simulink model "LETS_GOOOOOO"  (R2020b)
settings: Solver=VariableStepAuto  StartTime=0.0  StopTime=60  RelTol=1e-3
values from neighbouring files (symbols this model uses):
  A_2 = zeros(3)    [MPC_tune.m]
  B_2 = I_inv    [MPC_tune.m]
  C_2 = eye(3)    [MPC_tune.m]
  D_2 = zeros(3)    [MPC_tune.m]
  I_inv = inv(I_mat)    [MPC_tune.m]
  m = 941.102    [Linear_tuning.m]
  TcgCatia = [1 0 0 ... (first row only)    [MPC_tune.m]
undefined symbols (not defined in the file or in its folder): A_kal, B_kal, C_kal, Continuous, D_kal, delta_time, F_tot_max, Fb1_l, Fb1_u, Fb2_l, Fb2_u, Fb3_l, Fb3_u, Fb4_l, Fb4_u, Fc1_l, Fc1_u, Fc2_l, Fc2_u, Fc3_l, Fc3_u, fprop, Ft1_l, Ft1_u, Ft2_l, Ft2_u, Ft3_l, Ft3_u, Ft4_l, Ft4_u, g, r_0, r_cgCatia, r_trajectory, rho, T, t_finalgust, theta0, time, Time, time_delay, Tzy_Shard, u0_final, u0_ini, u1_final, u1_ini, u2_final, u2_ini, u_0, u_1, u_2, v_0, ZI_Cx, ZI_Cy, ZI_Cz, ZI_p, ZI_q, ZI_r
libraries: dspsigops x11, simulink x6, pid_lib x6, fuzblock x3, sharedutil x1, mpclib x1, dspmathops x1, ctrlSharedLib x1
(part 1 of 2)
settings Model: Creator=Jonathan van Zyl  LastModifiedBy=Jonathan van Zyl

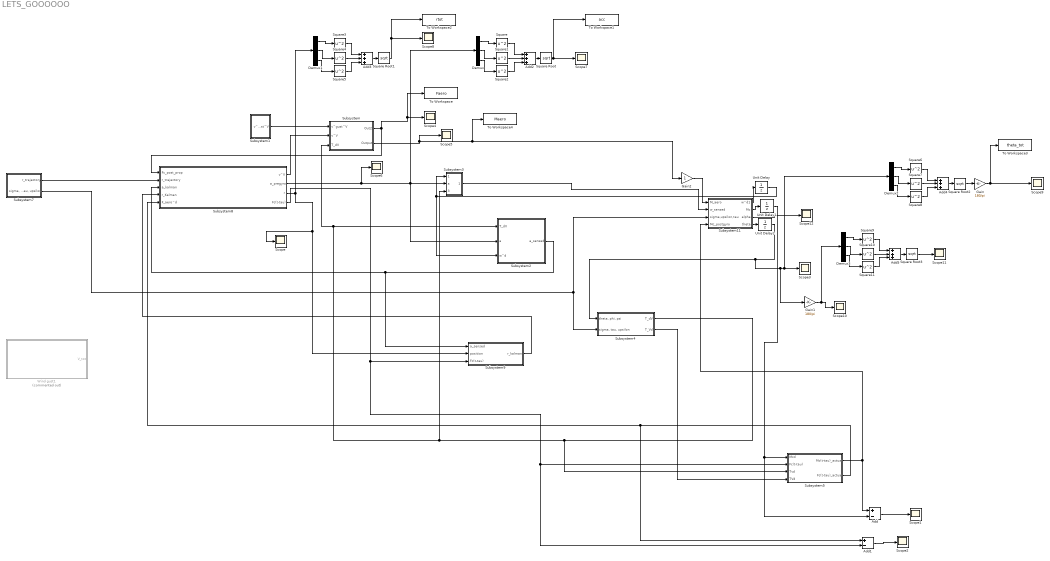
== system LETS_GOOOOOO ==
  Add : Sum  Inputs=+-
  Add1 : Sum  Inputs=+-
  Add{2..5} (4 alike) : Sum  Inputs=+++
  Demux{,1..3} (4 alike) : Demux  Outputs=3
  Gain : Gain  Gain=180/pi
  Gain1 : Gain  Gain=180/pi
  Gain2 : Gain
  Scope{,1..12} (13 alike) : Scope
  Square{,1..11} (12 alike) : Math  Operator=square  SaturateOnIntegerOverflow=on
  Square Root{,1..3} (4 alike) : Sqrt  SaturateOnIntegerOverflow=on
  Subsystem : Subsystem
  Subsystem1 : Subsystem
  Subsystem11 : Subsystem
  Subsystem2 : Subsystem
  Subsystem3 : Subsystem
  Subsystem4 : Subsystem
  Subsystem5 : Subsystem
  Subsystem7 : Subsystem
  Subsystem8 : Subsystem
  Subsystem9 : Subsystem
  To Workspace : ToWorkspace  VariableName=Faero  SaveFormat=Timeseries  SampleTime=-1
  To Workspace1 : ToWorkspace  VariableName=acc  SaveFormat=Timeseries  SampleTime=-1
  To Workspace2 : ToWorkspace  VariableName=rtot  SaveFormat=Timeseries  SampleTime=-1
  To Workspace3 : ToWorkspace  VariableName=theta_tot  SaveFormat=Timeseries  SampleTime=-1
  To Workspace4 : ToWorkspace  VariableName=Maero  SaveFormat=Timeseries  SampleTime=-1
  Unit Delay : UnitDelay  SampleTime=-1  HasFrameUpgradeWarning=on
  Unit Delay1 : UnitDelay  SampleTime=-1  HasFrameUpgradeWarning=on
  Unit Delay2 : UnitDelay  SampleTime=-1  HasFrameUpgradeWarning=on
  Wind gust1 : Subsystem  Commented=on
  wires:
  Unit Delay2/1 -> Gain1/1, Demux2/1, Scope3/1, Subsystem4/1("theta, phi, psi")
  Square9/1 -> Add5/1
  Subsystem/1(Out2) -> To Workspace/1, Scope4/1, Subsystem8/1(Fc_post_prop)
  Square1/1 -> Add2/2
  Subsystem/2(Output) -> Scope5/1, Gain2/1, To Workspace4/1
  Demux3/1 -> Square9/1
  Subsystem5/2(Fc(t-tau)_actual) -> Add1/1, Subsystem8/5(F_aero^d)
  Subsystem4/2(T_Vd) -> Subsystem5/4(TVd)
  Demux2/3 -> Square8/1
  Add1/1 -> Scope2/1
  Demux/3 -> Square2/1
  Square Root1/1 -> To Workspace2/1, Scope8/1
  Subsystem7/1(r_trajectory) -> Subsystem8/2(r_trajectory)
  Demux1/3 -> Square5/1
  Subsystem11/3(alpha) -> Scope12/1
  Demux2/2 -> Square7/1
  Subsystem8/2(a_pregyro) -> Scope6/1, Demux/1, Subsystem3/2(a), Subsystem2/2(a)
  Square10/1 -> Add5/2
  Add2/1 -> Square Root/1
  Subsystem5/1(Mc(t-tau)_actual) -> Subsystem11/4(Mc_postgyro), Add/1
  Demux/1 -> Square/1
  Square Root/1 -> To Workspace1/1, Scope7/1
  Subsystem7/2("sigma, tau, upsilon") -> Subsystem11/3(sigma,upsilon,tau), Subsystem4/2("sigma, tau, upsilon")
  Square4/1 -> Add3/2
  Subsystem4/1(T_dV) -> Subsystem5/3(Tvd), Subsystem/3(T_dV), Subsystem2/1(T_dV), Subsystem3/3(T_dV)
  Add4/1 -> Square Root2/1
  Unit Delay/1 -> Subsystem2/3(w^d), Subsystem3/1(w^d)
  Gain/1 -> To Workspace3/1, Scope9/1
  Demux2/1 -> Square6/1
  Subsystem2/1(a_sensed) -> Subsystem8/3(a_kalman), Subsystem9/1(a_sensed)
  Subsystem9/1(r_kalman) -> Subsystem8/4(r_Kalman)
  Square/1 -> Add2/1
  Square5/1 -> Add3/3
  Add/1 -> Scope1/1
  Demux/2 -> Square1/1
  Square6/1 -> Add4/1
  Square Root2/1 -> Gain/1
  Demux1/2 -> Square4/1
  Unit Delay1/1 -> Add/2, Subsystem5/1(Mcd)
  Square3/1 -> Add3/1
  Add3/1 -> Square Root1/1
  Subsystem8/3(r) -> Scope/1, Subsystem9/2(position), Demux1/1
  Demux1/1 -> Square3/1
  Square8/1 -> Add4/3
  Gain1/1 -> Demux3/1, Scope10/1
  Gain2/1 -> Subsystem11/1(M_aero)
  Demux3/2 -> Square10/1
  Subsystem8/1(v^V) -> Subsystem/2(v^V)
  Subsystem8/4(Fc(t-tau)) -> Add1/2, Subsystem5/2(Fc(t-tau)), Subsystem9/3(Fc(t-tau))
  Square7/1 -> Add4/2
  Square2/1 -> Add2/3
  Subsystem3/1(w^d1) -> Subsystem11/2(w_sensed)
  Add5/1 -> Square Root3/1
  Subsystem1/1(v^gust^V) -> Subsystem/1(v^gust^V)
  Square11/1 -> Add5/3
  Square Root3/1 -> Scope11/1
  Demux3/3 -> Square11/1
  Subsystem11/1(w^d1) -> Unit Delay/1
  Subsystem11/2(Mc) -> Unit Delay1/1
  Subsystem11/4(theta) -> Unit Delay2/1

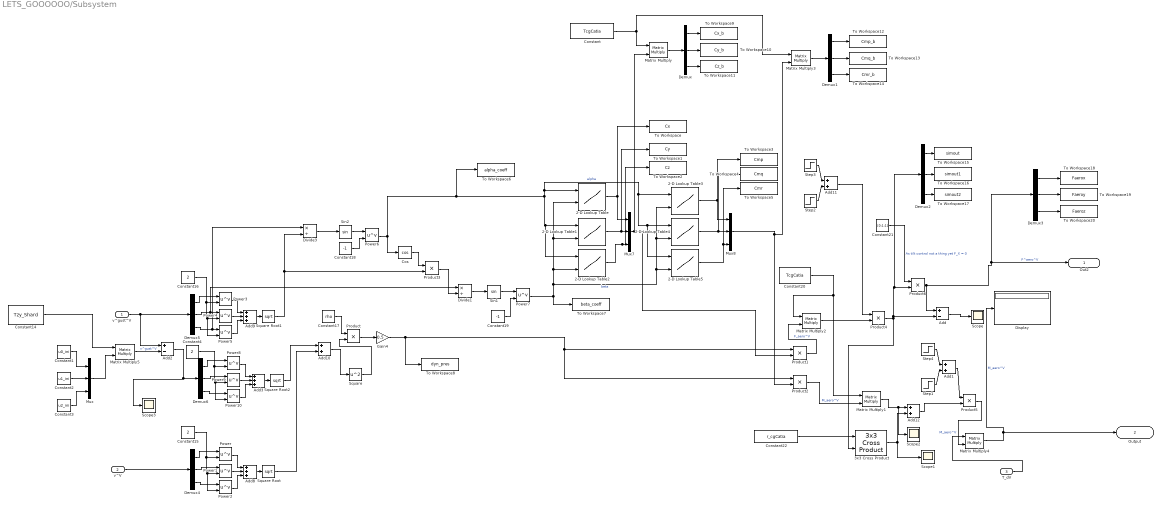
== system LETS_GOOOOOO/Subsystem ==
  v^gust^V : Inport
  v^V : Inport  Port=2
  T_dV : Inport  Port=3
  2-D Lookup Table : Lookup_n-D  BreakpointsForDimension1=[-180:1:180]  BreakpointsForDimension2=[-90:1:90]  Table=ZI_Cx  InternalRulePriority=Speed  RndMeth=Simplest  InputSameDT=on
      settings: InputPortMap=u0,u1
  2-D Lookup Table1 : Lookup_n-D  BreakpointsForDimension1=[-180:1:180]  BreakpointsForDimension2=[-90:1:90]  Table=ZI_Cy  InternalRulePriority=Speed  RndMeth=Simplest  InputSameDT=on
      settings: InputPortMap=u0,u1
  2-D Lookup Table2 : Lookup_n-D  BreakpointsForDimension1=[-180:1:180]  BreakpointsForDimension2=[-90:1:90]  Table=ZI_Cz  InternalRulePriority=Speed  RndMeth=Simplest  InputSameDT=on
      settings: InputPortMap=u0,u1
  2-D Lookup Table3 : Lookup_n-D  BreakpointsForDimension1=[-180:1:180]  BreakpointsForDimension2=[-90:1:90]  Table=ZI_p  InternalRulePriority=Speed  RndMeth=Simplest  InputSameDT=on
      settings: InputPortMap=u0,u1
  2-D Lookup Table4 : Lookup_n-D  BreakpointsForDimension1=[-180:1:180]  BreakpointsForDimension2=[-90:1:90]  Table=ZI_q  InternalRulePriority=Speed  RndMeth=Simplest  InputSameDT=on
      settings: InputPortMap=u0,u1
  2-D Lookup Table5 : Lookup_n-D  BreakpointsForDimension1=[-180:1:180]  BreakpointsForDimension2=[-90:1:90]  Table=ZI_r  InternalRulePriority=Speed  RndMeth=Simplest  InputSameDT=on
      settings: InputPortMap=u0,u1
  3x3 Cross Product : sharedutil/3x3 Cross Product  aMode=aMode
      settings: SourceProductBaseCode=AE,PW,MT,UV,VE,VP
  Add : Sum  Inputs=+-
  Add{1,10..12} (4 alike) : Sum
  Add2 : Sum  Inputs=+-
  Add3 : Sum  Inputs=+++
  Add8 : Sum  Inputs=+++
  Add9 : Sum  Inputs=+++
  Constant : Constant  Value=TcgCatia
  Constant1 : Constant  Value=u0_ini
  Constant14 : Constant  Value=Tzy_Shard
  Constant15 : Constant  Value=2
  Constant16 : Constant  Value=2
  Constant17 : Constant  Value=rho
  Constant18 : Constant  Value=-1
  Constant19 : Constant  Value=-1
  Constant2 : Constant  Value=u1_ini
  Constant20 : Constant  Value=TcgCatia
  Constant21 : Constant  Value=[0;1;1]
  Constant22 : Constant  Value=r_cgCatia
  Constant3 : Constant  Value=u2_ini
  Constant4 : Constant  Value=2
  Cos : Trigonometry  Operator=cos
  Demux{,1..6} (7 alike) : Demux  Outputs=3
  Display : Display
  Divide1 : Product  Inputs=*/
  Divide3 : Product  Inputs=*/
  Gain4 : Gain  Gain=0.5
  Matrix Multiply{,1..5} (6 alike) : Product  Multiplication=Matrix(*)
  Mux : Mux  Inputs=3
  Mux7 : Mux  Inputs=3
  Mux8 : Mux  Inputs=3
  Power{,1..10} (11 alike) : Math  Operator=pow  SaturateOnIntegerOverflow=on
  Product{,1..6} (7 alike) : Product
  Scope{,1..3} (4 alike) : Scope
  Sin1 : Trigonometry
  Sin2 : Trigonometry
  Square : Math  Operator=square  SaturateOnIntegerOverflow=on
  Square Root : Sqrt  SaturateOnIntegerOverflow=on
  Square Root1 : Sqrt  SaturateOnIntegerOverflow=on
  Square Root2 : Sqrt  SaturateOnIntegerOverflow=on
  Step1 : Step  Time=0  SampleTime=0
  Step2 : Step  Time=0  SampleTime=0
  Step3 : Step  Time=time  After=-1  SampleTime=0
  Step4 : Step  Time=time  After=-1  SampleTime=0
  To Workspace : ToWorkspace  VariableName=Cx  SaveFormat=Timeseries  SampleTime=-1
  To Workspace1 : ToWorkspace  VariableName=Cy  SaveFormat=Timeseries  SampleTime=-1
  To Workspace10 : ToWorkspace  VariableName=Cy_b  SaveFormat=Timeseries  SampleTime=-1
  To Workspace11 : ToWorkspace  VariableName=Cz_b  SaveFormat=Timeseries  SampleTime=-1
  To Workspace12 : ToWorkspace  VariableName=Cmp_b  SaveFormat=Timeseries  SampleTime=-1
  To Workspace13 : ToWorkspace  VariableName=Cmq_b  SaveFormat=Timeseries  SampleTime=-1
  To Workspace14 : ToWorkspace  VariableName=Cmr_b  SaveFormat=Timeseries  SampleTime=-1
  To Workspace15 : ToWorkspace  VariableName=simout  SaveFormat=Timeseries  SampleTime=-1
  To Workspace16 : ToWorkspace  VariableName=simout1  SaveFormat=Timeseries  SampleTime=-1
  To Workspace17 : ToWorkspace  VariableName=simout2  SaveFormat=Timeseries  SampleTime=-1
  To Workspace18 : ToWorkspace  VariableName=Faerox  SaveFormat=Timeseries  SampleTime=-1
  To Workspace19 : ToWorkspace  VariableName=Faeroy  SaveFormat=Timeseries  SampleTime=-1
  To Workspace2 : ToWorkspace  VariableName=Cz  SaveFormat=Timeseries  SampleTime=-1
  To Workspace20 : ToWorkspace  VariableName=Faeroz  SaveFormat=Timeseries  SampleTime=-1
  To Workspace3 : ToWorkspace  VariableName=Cmp  SaveFormat=Timeseries  SampleTime=-1
  To Workspace4 : ToWorkspace  VariableName=Cmq  SaveFormat=Timeseries  SampleTime=-1
  To Workspace5 : ToWorkspace  VariableName=Cmr  SaveFormat=Timeseries  SampleTime=-1
  To Workspace6 : ToWorkspace  VariableName=alpha_coeff  SaveFormat=Timeseries  SampleTime=-1
  To Workspace7 : ToWorkspace  VariableName=beta_coeff  SaveFormat=Timeseries  SampleTime=-1
  To Workspace8 : ToWorkspace  VariableName=dyn_pres  SaveFormat=Timeseries  SampleTime=-1
  To Workspace9 : ToWorkspace  VariableName=Cx_b  SaveFormat=Timeseries  SampleTime=-1
  Out2 : Outport
  Output : Outport  Port=2
  wires:
  Demux5/1 -> Power3/1
  Constant21/1 -> Product6/1  "As tilt control not a thing yet F_X = 0"
  2-D Lookup Table3/1 -> To Workspace3/1, Mux8/1
  Constant17/1 -> Product/1
  Power5/1 -> Add9/3
  Product4/1 -> Demux2/1, Product6/2, Add/2, 3x3 Cross Product/2
  Power7/1 -> 2-D Lookup Table/2, 2-D Lookup Table1/2, 2-D Lookup Table2/2, 2-D Lookup Table3/2, 2-D Lookup Table4/2, 2-D Lookup Table5/2, To Workspace7/1  "beta"
  2-D Lookup Table2/1 -> To Workspace2/1, Mux7/3
  Power3/1 -> Add9/1
  Constant15/1 -> Power2/2, Power1/2, Power/2
  Sin1/1 -> Power7/1
  Square/1 -> Product/2
  Demux4/2 -> Power1/1
  Gain4/1 -> To Workspace8/1, Product2/1, Product1/1
  Square Root1/1 -> Product3/2, Divide3/2
  Product1/1 -> Matrix Multiply2/2  "F_aero^V"
  2-D Lookup Table1/1 -> To Workspace1/1, Mux7/2
  Add8/1 -> Square Root/1
  Cos/1 -> Product3/1
  3x3 Cross Product/1 -> Add12/2, Scope1/1
  Power2/1 -> Add8/3
  Add9/1 -> Square Root1/1
  Divide3/1 -> Sin2/1
  Mux7/1 -> Matrix Multiply/2, Product1/2
  Demux5/2 -> Divide1/1, Power4/1
  Product3/1 -> Divide1/2
  Constant22/1 -> 3x3 Cross Product/1
  Product2/1 -> Matrix Multiply1/2  "M_aero^V"
  Demux4/3 -> Power2/1
  Square Root/1 -> Add10/2
  Constant16/1 -> Power5/2, Power4/2, Power3/2
  2-D Lookup Table5/1 -> To Workspace5/1, Mux8/3
  v^gust^V/1 -> Add2/1, Demux5/1
  Divide1/1 -> Sin1/1
  Power1/1 -> Add8/2
  Constant20/1 -> Matrix Multiply1/1, Matrix Multiply2/1
  Power4/1 -> Add9/2
  Power/1 -> Add8/1
  2-D Lookup Table4/1 -> To Workspace4/1, Mux8/2
  Matrix Multiply1/1 -> Scope2/1, Add12/1
  Mux8/1 -> Matrix Multiply3/2, Product2/2
  Constant18/1 -> Power6/2
  Demux4/1 -> Power/1
  Product6/1 -> Add/1, Out2/1, Demux3/1  "F^aero^V"
  Demux5/3 -> Divide3/1, Power5/1
  Product/1 -> Gain4/1
  Power6/1 -> Cos/1, To Workspace6/1, 2-D Lookup Table/1, 2-D Lookup Table5/1, 2-D Lookup Table4/1, 2-D Lookup Table3/1, 2-D Lookup Table2/1, 2-D Lookup Table1/1  "alpha"
  Sin2/1 -> Power6/1
  Constant19/1 -> Power7/2
  2-D Lookup Table/1 -> Mux7/1, To Workspace/1
  Add10/1 -> Square/1
  Matrix Multiply4/1 -> Display/1, Output/1  "M_aero^V"
  T_dV/1 -> Matrix Multiply4/1
  v^V/1 -> Demux4/1
  Add/1 -> Scope/1
  Constant/1 -> Matrix Multiply3/1, Matrix Multiply/1
  Matrix Multiply/1 -> Demux/1
  Demux/1 -> To Workspace9/1
  Demux/2 -> To Workspace10/1
  Demux/3 -> To Workspace11/1
  Matrix Multiply3/1 -> Demux1/1
  Demux1/1 -> To Workspace12/1
  Demux1/2 -> To Workspace13/1
  Demux1/3 -> To Workspace14/1
  Demux2/1 -> To Workspace15/1
  Demux2/2 -> To Workspace16/1
  Demux2/3 -> To Workspace17/1
  Demux3/1 -> To Workspace18/1
  Demux3/2 -> To Workspace19/1
  Demux3/3 -> To Workspace20/1
  Step3/1 -> Add11/1
  Add11/1 -> Product4/1
  Step2/1 -> Add11/2
  Matrix Multiply2/1 -> Product4/2
  Add1/1 -> Product5/1
  Step1/1 -> Add1/2
  Step4/1 -> Add1/1
  Product5/1 -> Matrix Multiply4/2  "M_aero^V"
  Add12/1 -> Product5/2
  Mux/1 -> Matrix Multiply5/2
  Constant3/1 -> Mux/3
  Constant1/1 -> Mux/1
  Constant2/1 -> Mux/2
  Add2/1 -> Demux6/1, Scope3/1
  Constant14/1 -> Matrix Multiply5/1
  Matrix Multiply5/1 -> Add2/2  "v^gust^V"
  Power10/1 -> Add3/3
  Demux6/3 -> Power10/1
  Add3/1 -> Square Root2/1
  Power9/1 -> Add3/2
  Power8/1 -> Add3/1
  Demux6/2 -> Power9/1
  Demux6/1 -> Power8/1
  Square Root2/1 -> Add10/1
  Constant4/1 -> Power8/2, Power9/2, Power10/2

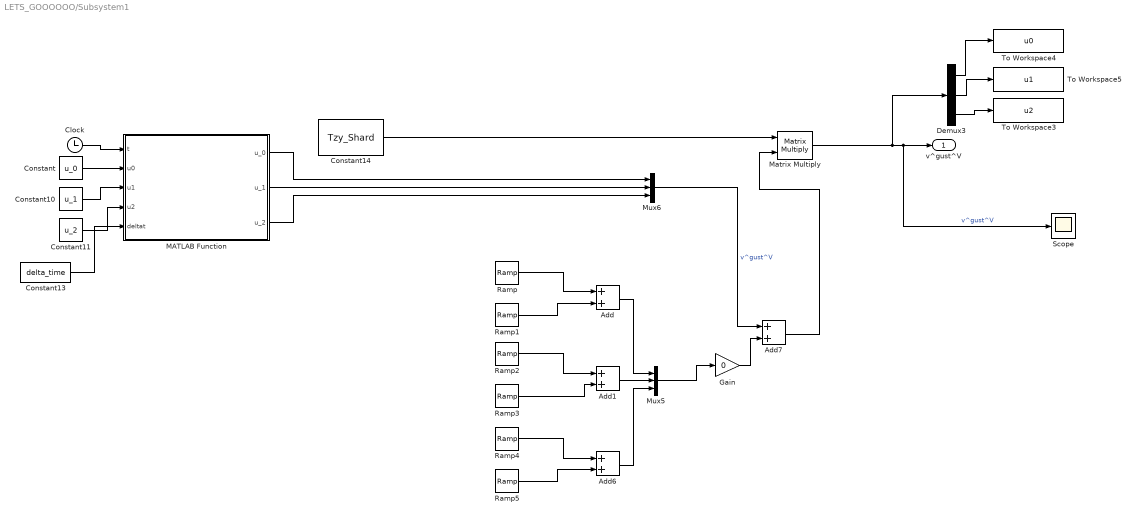
== system LETS_GOOOOOO/Subsystem1 ==
  Add{,1,6..7} (4 alike) : Sum
  Clock : Clock
  Constant : Constant  Value=u_0
  Constant10 : Constant  Value=u_1
  Constant11 : Constant  Value=u_2
  Constant13 : Constant  Value=delta_time
  Constant14 : Constant  Value=Tzy_Shard
  Demux3 : Demux  Outputs=3
  Gain : Gain  Gain=0
  MATLAB Function : MATLAB Function  TreatAsAtomicUnit=on
  Matrix Multiply : Product  Multiplication=Matrix(*)
  Mux5 : Mux  Inputs=3
  Mux6 : Mux  Inputs=3
  Ramp : simulink/Sources/Ramp  slope=-1  start=t_finalgust  InitialOutput=0
  Ramp1 : simulink/Sources/Ramp  slope=1  start=t_finalgust + u0_final  InitialOutput=0
  Ramp2 : simulink/Sources/Ramp  slope=-1  start=t_finalgust  InitialOutput=0
  Ramp3 : simulink/Sources/Ramp  slope=1  start=t_finalgust + u1_final  InitialOutput=0
  Ramp4 : simulink/Sources/Ramp  slope=-1  start=t_finalgust  InitialOutput=0
  Ramp5 : simulink/Sources/Ramp  slope=1  start=t_finalgust + u2_final  InitialOutput=0
  Scope : Scope
  To Workspace3 : ToWorkspace  VariableName=u2  SaveFormat=Timeseries  SampleTime=-1
  To Workspace4 : ToWorkspace  VariableName=u0  SaveFormat=Timeseries  SampleTime=-1
  To Workspace5 : ToWorkspace  VariableName=u1  SaveFormat=Timeseries  SampleTime=-1
  v^gust^V : Outport
  wires:
  Add1/1 -> Mux5/2
  MATLAB Function/1(u_0) -> Mux6/1
  Add7/1 -> Matrix Multiply/2
  Constant13/1 -> MATLAB Function/5(deltat)
  Ramp4/1 -> Add6/1
  Ramp3/1 -> Add1/2
  Constant11/1 -> MATLAB Function/4(u2)
  Constant/1 -> MATLAB Function/2(u0)
  Ramp1/1 -> Add/2
  Mux5/1 -> Gain/1
  Constant14/1 -> Matrix Multiply/1
  MATLAB Function/2(u_1) -> Mux6/2
  Constant10/1 -> MATLAB Function/3(u1)
  Ramp/1 -> Add/1
  Matrix Multiply/1 -> Demux3/1, Scope/1, v^gust^V/1  "v^gust^V"
  Ramp5/1 -> Add6/2
  Add6/1 -> Mux5/3
  Clock/1 -> MATLAB Function/1(t)
  MATLAB Function/3(u_2) -> Mux6/3
  Add/1 -> Mux5/1
  Ramp2/1 -> Add1/1
  Mux6/1 -> Add7/1  "v^gust^V"
  Demux3/3 -> To Workspace3/1
  Demux3/2 -> To Workspace5/1
  Demux3/1 -> To Workspace4/1
  Gain/1 -> Add7/2

== system LETS_GOOOOOO/Subsystem11 ==
  M_aero : Inport
  w_sensed : Inport  Port=2
  sigma,upsilon,tau : Inport  Port=3
  Mc_postgyro : Inport  Port=4
  Add : Sum  Inputs=+++
  Demux : Demux  Outputs=3
  Gain3 : Gain  Gain=180/pi
  Scope : Scope
  Scope1 : Scope
  Scope8 : Scope
  Square : Math  Operator=square  SaturateOnIntegerOverflow=on
  Square Root : Sqrt  SaturateOnIntegerOverflow=on
  Square1 : Math  Operator=square  SaturateOnIntegerOverflow=on
  Square2 : Math  Operator=square  SaturateOnIntegerOverflow=on
  Subsystem : Subsystem
  To Workspace : ToWorkspace  VariableName=angle_deg  SaveFormat=Timeseries  SampleTime=-1
  To Workspace1 : ToWorkspace  VariableName=alpha  SaveFormat=Timeseries  SampleTime=-1
  initial w : Constant  Value=[0;0;0]
  w^d1 : Outport
  Mc : Outport  Port=2
  alpha : Outport  Port=3
  theta : Outport  Port=4
  wires:
  Mc_postgyro/1 -> Subsystem/5(Mcpost)
  Subsystem/4(alpha) -> Demux/1, Scope/1, alpha/1
  Demux/1 -> Square/1
  Demux/2 -> Square1/1
  Demux/3 -> Square2/1
  Square/1 -> Add/1
  Square1/1 -> Add/2
  Square2/1 -> Add/3
  Add/1 -> Square Root/1
  Square Root/1 -> To Workspace1/1, Scope1/1
  sigma,upsilon,tau/1 -> Subsystem/3(sigma,tau,upsilon)
  initial w/1 -> Subsystem/4(initial w)
  M_aero/1 -> Subsystem/2(M_aero)
  Subsystem/3(Mc) -> Mc/1
  Subsystem/2(w_out) -> w^d1/1
  Subsystem/1(theta_out) -> Gain3/1, theta/1
  Gain3/1 -> To Workspace/1, Scope8/1
  w_sensed/1 -> Subsystem/1(w_sensed)

== system LETS_GOOOOOO/Subsystem2 ==
  T_dV : Inport
  a : Inport  Port=2
  w^d : Inport  Port=3
  Display1 : Display
  Display2 : Display
  MATLAB Function1 : MATLAB Function  Commented=on  TreatAsAtomicUnit=on
  Terminator5 : Terminator
  Terminator6 : Terminator
  Transpose1 : Math  Operator=transpose  SaturateOnIntegerOverflow=on
  Transpose2 : Math  Operator=transpose  SaturateOnIntegerOverflow=on
  Transpose3 : Math  Operator=transpose  SaturateOnIntegerOverflow=on
  a_sensed : Outport
  wires:
  a/1 -> Transpose1/1
  Transpose1/1 -> Display1/1, Transpose2/1, Display2/1  "a_sensed"
  Transpose3/1 -> Terminator5/1
  T_dV/1 -> Terminator6/1
  Transpose2/1 -> a_sensed/1  "a_sensed"
  w^d/1 -> Transpose3/1

== system LETS_GOOOOOO/Subsystem3 ==
  w^d : Inport
  a : Inport  Port=2
  T_dV : Inport  Port=3
  Add : Sum  Inputs=+-
  Add1 : Sum
  Demux21 : Demux  Outputs=3
  Demux22 : Demux  Outputs=3
  Gain : Gain  Gain=0
  Gain1 : Gain
  MATLAB Function10 : MATLAB Function  TreatAsAtomicUnit=on
  Matrix Multiply4 : Product  Multiplication=Matrix(*)
  Mux14 : Mux  Inputs=3
  To Workspace : ToWorkspace  VariableName=gyro  SaveFormat=Timeseries  SampleTime=-1
  w^d1 : Outport
  wires:
  Demux21/3 -> MATLAB Function10/3(zvel)
  Demux22/1 -> MATLAB Function10/4(accx)
  Demux22/2 -> MATLAB Function10/5(accy)
  Demux22/3 -> MATLAB Function10/6(accz)
  MATLAB Function10/1(wx) -> Mux14/1
  Demux21/1 -> MATLAB Function10/1(xvel)
  MATLAB Function10/2(wy) -> Mux14/2
  Demux21/2 -> MATLAB Function10/2(yvel)
  MATLAB Function10/3(wz) -> Mux14/3
  Matrix Multiply4/1 -> Demux22/1
  Mux14/1 -> Gain/1, Add/2  "w^d"
  T_dV/1 -> Matrix Multiply4/1
  a/1 -> Matrix Multiply4/2
  w^d/1 -> Gain1/1, Add/1, Demux21/1
  Add/1 -> To Workspace/1
  Gain/1 -> Add1/1
  Gain1/1 -> Add1/2
  Add1/1 -> w^d1/1

== system LETS_GOOOOOO/Subsystem4 ==
  "theta, phi, psi" : Inport
  "sigma, tau, upsilon" : Inport  Port=2
  Demux6 : Demux  Outputs=3
  Demux7 : Demux  Outputs=3
  MATLAB Function2 : MATLAB Function  TreatAsAtomicUnit=on
  MATLAB Function3 : MATLAB Function  TreatAsAtomicUnit=on
  Matrix Multiply7 : Product  Multiplication=Matrix(*)
  Terminator{7..10} (4 alike) : Terminator
  Transpose4 : Math  Operator=transpose  SaturateOnIntegerOverflow=on
  Transpose5 : Math  Operator=transpose  SaturateOnIntegerOverflow=on
  Transpose6 : Math  Operator=transpose  SaturateOnIntegerOverflow=on
  T_dV : Outport
  T_Vd : Outport  Port=2
  wires:
  Matrix Multiply7/1 -> T_Vd/1, Transpose6/1  "T_Vd"
  Demux7/1 -> MATLAB Function3/1(theta_x)
  "theta, phi, psi"/1 -> Demux6/1
  Demux6/3 -> MATLAB Function2/3(theta_z)
  Demux7/3 -> MATLAB Function3/3(theta_z)
  "sigma, tau, upsilon"/1 -> Demux7/1
  Demux6/1 -> MATLAB Function2/1(theta_x)
  Transpose5/1 -> Terminator9/1, Matrix Multiply7/2  "T_Vt"
  MATLAB Function2/1(Transformation_Mat) -> Terminator7/1, Transpose4/1  "T_dt"
  Transpose4/1 -> Terminator8/1, Matrix Multiply7/1  "T_td"
  MATLAB Function3/1(Transformation_Mat) -> Terminator10/1, Transpose5/1  "T_tV"
  Demux6/2 -> MATLAB Function2/2(theta_y)
  Demux7/2 -> MATLAB Function3/2(theta_y)
  Transpose6/1 -> T_dV/1  "T_dV"

== system LETS_GOOOOOO/Subsystem5 ==
  Mcd : Inport
  Fc(t-tau) : Inport  Port=2
  Tvd : Inport  Port=3
  TVd : Inport  Port=4
  Gain6 : Gain
  MATLAB Function4 : MATLAB Function  Commented=on  TreatAsAtomicUnit=on
  MATLAB Function5 : MATLAB Function  Commented=on  TreatAsAtomicUnit=on
  Matrix Multiply5 : Product  Multiplication=Matrix(*)
  Scope16 : Scope
  Scope17 : Scope
  Scope18 : Scope
  Subsystem : Subsystem
  Subsystem1 : Subsystem
  Subsystem2 : Subsystem
  Subsystem3 : Subsystem
  Subsystem4 : Subsystem
  Turn off for PID tune : Gain
  Mc(t-tau)_actual : Outport
  Fc(t-tau)_actual : Outport  Port=2
  wires:
  Mcd/1 -> Gain6/1
  Turn off for PID tune/1 -> Matrix Multiply5/2
  Tvd/1 -> Matrix Multiply5/1
  Fc(t-tau)/1 -> Turn off for PID tune/1
  MATLAB Function5/1(F1) -> MATLAB Function4/1(F1)
  MATLAB Function5/3(F3) -> MATLAB Function4/3(F3)
  MATLAB Function5/2(F2) -> MATLAB Function4/2(F2)
  Matrix Multiply5/1 -> Subsystem/1(F_c_d)  "F_c_d"
  Gain6/1 -> Subsystem/2(M_c_d)  "M_c_d"
  Subsystem/1(Fb_wanted) -> Subsystem1/1(In1)
  Subsystem/2(Ft_wanted) -> Subsystem1/2(In2)
  Subsystem/3(Fc_wanted) -> Subsystem1/3(In3)
  Subsystem1/1(Out1) -> Subsystem2/1(In1)
  Subsystem1/2(Out2) -> Subsystem2/2(In2)
  Subsystem1/3(Out3) -> Subsystem2/3(In3)
  Subsystem3/1(Out1) -> Scope17/1, Subsystem4/2(In2)
  Subsystem2/1(F_c_max) -> Subsystem3/1(In1)
  Subsystem2/2(F_t_max) -> Subsystem3/2(In2)
  Subsystem2/3(Out3) -> Subsystem3/3(In3)
  Subsystem2/4(Out4) -> Subsystem3/4(Ft3)
  Subsystem2/5(Out5) -> Subsystem3/5(Ft4)
  Subsystem2/6(Out6) -> Subsystem3/6(Fb1)
  Subsystem2/7(Out7) -> Subsystem3/7(In7)
  Subsystem2/8(Out8) -> Subsystem3/8(Fb3)
  Subsystem2/9(Out9) -> Subsystem3/9(In9)
  Subsystem3/2(Mc(t-tau)_actual) -> Mc(t-tau)_actual/1
  Subsystem4/1(Fc(t-tau)_actual) -> Scope16/1, Fc(t-tau)_actual/1
  TVd/1 -> Subsystem4/1(TVd)
  Subsystem4/2(Fc(t-tau)_actual1) -> Scope18/1

== system LETS_GOOOOOO/Subsystem7 ==
  Constant2 : Constant  Value=r_trajectory
  Constant9 : Constant  Value=[0;0;0]
  r_trajectory : Outport
  "sigma, tau, upsilon" : Outport  Port=2
  wires:
  Constant2/1 -> r_trajectory/1
  Constant9/1 -> "sigma, tau, upsilon"/1  "sigma, tau, upsilon"

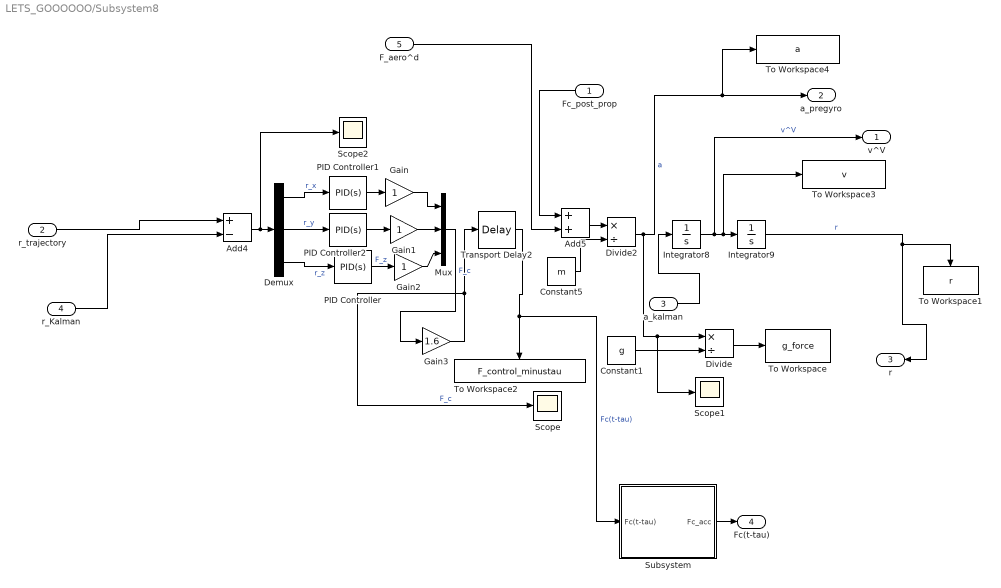
== system LETS_GOOOOOO/Subsystem8 ==
  Fc_post_prop : Inport
  r_trajectory : Inport  Port=2
  a_kalman : Inport  Port=3
  r_Kalman : Inport  Port=4
  F_aero^d : Inport  Port=5
  Add4 : Sum  Inputs=+-
  Add5 : Sum
  Constant1 : Constant  Value=g
  Constant5 : Constant  Value=m
  Demux : Demux  Outputs=3
  Divide : Product  Inputs=*/
  Divide2 : Product  Inputs=*/
  Gain : Gain
  Gain1 : Gain
  Gain2 : Gain
  Gain3 : Gain  Gain=1.6
  Integrator8 : Integrator  InitialCondition=v_0
  Integrator9 : Integrator  InitialCondition=r_0
  Mux : Mux  Inputs=3
  PID Controller : pid_lib/PID Controller  Controller=PID  Form=Parallel  TimeDomain=Continuous-time  UseExternalTs=off  SampleTime=-1  IntegratorMethod=Forward Euler  FilterMethod=Forward Euler  ControllerParametersSource=internal  P=160.734193661502  I=6.85755125615993  D=923.025793270617  UseFilter=on  N=10.4897155810233  TunerSelectOption=Transfer Function Based (PID Tuner App)  InitialConditionSource=internal  InitialConditionForIntegrator=0  InitialConditionForFilter=0  DifferentiatorICPrevScaledInput=0  ExternalReset=none  TrackingMode=off  Kt=1  LimitOutput=off  SatLimitsSource=internal  UpperSaturationLimit=inf  LowerSaturationLimit=-inf  LinearizeAsGain=on  AntiWindupMode=none  Kb=1  POutMin=[]  POutMax=[]  IOutMin=[]  IOutMax=[]  DOutMin=[]  DOutMax=[]  NOutMin=[]  NOutMax=[]  SumOutMin=[]  SumOutMax=[]  SaturationOutMin=[]  SaturationOutMax=[]  PParamMin=[]  PParamMax=[]  IParamMin=[]  IParamMax=[]  DParamMin=[]  DParamMax=[]  NParamMin=[]  NParamMax=[]  KbParamMin=[]  KbParamMax=[]  KtParamMin=[]  KtParamMax=[]  KbOutMin=[]  KbOutMax=[]  KtOutMin=[]  KtOutMax=[]  IntegratorOutMin=[]  IntegratorOutMax=[]  FilterOutMin=[]  FilterOutMax=[]  SumI1OutMin=[]  SumI1OutMax=[]  SumI2OutMin=[]  SumI2OutMax=[]  SumI3OutMin=[]  SumI3OutMax=[]  SumI4OutMin=[]  SumI4OutMax=[]  SumDOutMin=[]  SumDOutMax=[]  DifferentiatorOutMin=[]  DifferentiatorOutMax=[]  FilterDiffOutCoefMin=[]  FilterDiffOutCoefMax=[]  ReciprocalOutMin=[]  ReciprocalOutMax=[]  SumDenOutMin=[]  SumDenOutMax=[]  SumNumOutMin=[]  SumNumOutMax=[]  DivideOutMin=[]  DivideOutMax=[]  UdiffTsProdOutMin=[]  UdiffTsProdOutMax=[]  NTsProdOutMin=[]  NTsProdOutMax=[]  UintegralTsProdOutMin=[]  UintegralTsProdOutMax=[]  UngainTsProdOutMin=[]  UngainTsProdOutMax=[]  IntegratorContinuousStateAttributes=''  IntegratorStateMustResolveToSignalObject=off  IntegratorRTWStateStorageClass=Auto  FilterContinuousStateAttributes=''  FilterStateMustResolveToSignalObject=off  FilterRTWStateStorageClass=Auto  ParallelPVariant=InternalParameters  IdealPVariant=Disabled  IVariant=InternalParameters  DVariant=InternalParameters  IntegratorVariant=Continuous  SatVariant=Disabled  AWVariant=Passthrough  PCopyVariant=Disabled  TRVariant=Disabled  FdbkBlocksVariant=Forward  IdealPFdbkVariant=Disabled  SatFdbkVariant=Disabled  DerivativeFilterVariant=ContFilter  NVariant=InternalParameters  NCopyVariant=Disabled  FilterICVariant=InternalICsFilter  IntegratorICVariant=InternalICs  ExternalResetVariant=Disabled  TRSumVariant=Passthrough  SumFdbkVariant=Disabled  SumVariant=Sum_PID  TsampFilterVariant=InternalTs  TsampNgainVariant=Passthrough  TsampIntegralVariant=Passthrough  ExternalSaturationOutDataTypeStr=Inherit: Same as second input
  PID Controller1 : pid_lib/PID Controller  Controller=PID  Form=Parallel  TimeDomain=Continuous-time  UseExternalTs=off  SampleTime=-1  IntegratorMethod=Forward Euler  FilterMethod=Forward Euler  ControllerParametersSource=internal  P=160.734193661502  I=6.85755125615993  D=923.025793270617  UseFilter=on  N=10.4897155810233  TunerSelectOption=Transfer Function Based (PID Tuner App)  InitialConditionSource=internal  InitialConditionForIntegrator=0  InitialConditionForFilter=0  DifferentiatorICPrevScaledInput=0  ExternalReset=none  TrackingMode=off  Kt=1  LimitOutput=off  SatLimitsSource=internal  UpperSaturationLimit=inf  LowerSaturationLimit=-inf  LinearizeAsGain=on  AntiWindupMode=none  Kb=1  POutMin=[]  POutMax=[]  IOutMin=[]  IOutMax=[]  DOutMin=[]  DOutMax=[]  NOutMin=[]  NOutMax=[]  SumOutMin=[]  SumOutMax=[]  SaturationOutMin=[]  SaturationOutMax=[]  PParamMin=[]  PParamMax=[]  IParamMin=[]  IParamMax=[]  DParamMin=[]  DParamMax=[]  NParamMin=[]  NParamMax=[]  KbParamMin=[]  KbParamMax=[]  KtParamMin=[]  KtParamMax=[]  KbOutMin=[]  KbOutMax=[]  KtOutMin=[]  KtOutMax=[]  IntegratorOutMin=[]  IntegratorOutMax=[]  FilterOutMin=[]  FilterOutMax=[]  SumI1OutMin=[]  SumI1OutMax=[]  SumI2OutMin=[]  SumI2OutMax=[]  SumI3OutMin=[]  SumI3OutMax=[]  SumI4OutMin=[]  SumI4OutMax=[]  SumDOutMin=[]  SumDOutMax=[]  DifferentiatorOutMin=[]  DifferentiatorOutMax=[]  FilterDiffOutCoefMin=[]  FilterDiffOutCoefMax=[]  ReciprocalOutMin=[]  ReciprocalOutMax=[]  SumDenOutMin=[]  SumDenOutMax=[]  SumNumOutMin=[]  SumNumOutMax=[]  DivideOutMin=[]  DivideOutMax=[]  UdiffTsProdOutMin=[]  UdiffTsProdOutMax=[]  NTsProdOutMin=[]  NTsProdOutMax=[]  UintegralTsProdOutMin=[]  UintegralTsProdOutMax=[]  UngainTsProdOutMin=[]  UngainTsProdOutMax=[]  IntegratorContinuousStateAttributes=''  IntegratorStateMustResolveToSignalObject=off  IntegratorRTWStateStorageClass=Auto  FilterContinuousStateAttributes=''  FilterStateMustResolveToSignalObject=off  FilterRTWStateStorageClass=Auto  ParallelPVariant=InternalParameters  IdealPVariant=Disabled  IVariant=InternalParameters  DVariant=InternalParameters  IntegratorVariant=Continuous  SatVariant=Disabled  AWVariant=Passthrough  PCopyVariant=Disabled  TRVariant=Disabled  FdbkBlocksVariant=Forward  IdealPFdbkVariant=Disabled  SatFdbkVariant=Disabled  DerivativeFilterVariant=ContFilter  NVariant=InternalParameters  NCopyVariant=Disabled  FilterICVariant=InternalICsFilter  IntegratorICVariant=InternalICs  ExternalResetVariant=Disabled  TRSumVariant=Passthrough  SumFdbkVariant=Disabled  SumVariant=Sum_PID  TsampFilterVariant=InternalTs  TsampNgainVariant=Passthrough  TsampIntegralVariant=Passthrough  ExternalSaturationOutDataTypeStr=Inherit: Same as second input
  PID Controller2 : pid_lib/PID Controller  Controller=PID  Form=Parallel  TimeDomain=Continuous-time  UseExternalTs=off  SampleTime=-1  IntegratorMethod=Forward Euler  FilterMethod=Forward Euler  ControllerParametersSource=internal  P=160.734193661502*2  I=6.85755125615993  D=923.025793270617  UseFilter=on  N=10.4897155810233  TunerSelectOption=Transfer Function Based (PID Tuner App)  InitialConditionSource=internal  InitialConditionForIntegrator=0  InitialConditionForFilter=0  DifferentiatorICPrevScaledInput=0  ExternalReset=none  TrackingMode=off  Kt=1  LimitOutput=off  SatLimitsSource=internal  UpperSaturationLimit=inf  LowerSaturationLimit=-inf  LinearizeAsGain=on  AntiWindupMode=none  Kb=1  POutMin=[]  POutMax=[]  IOutMin=[]  IOutMax=[]  DOutMin=[]  DOutMax=[]  NOutMin=[]  NOutMax=[]  SumOutMin=[]  SumOutMax=[]  SaturationOutMin=[]  SaturationOutMax=[]  PParamMin=[]  PParamMax=[]  IParamMin=[]  IParamMax=[]  DParamMin=[]  DParamMax=[]  NParamMin=[]  NParamMax=[]  KbParamMin=[]  KbParamMax=[]  KtParamMin=[]  KtParamMax=[]  KbOutMin=[]  KbOutMax=[]  KtOutMin=[]  KtOutMax=[]  IntegratorOutMin=[]  IntegratorOutMax=[]  FilterOutMin=[]  FilterOutMax=[]  SumI1OutMin=[]  SumI1OutMax=[]  SumI2OutMin=[]  SumI2OutMax=[]  SumI3OutMin=[]  SumI3OutMax=[]  SumI4OutMin=[]  SumI4OutMax=[]  SumDOutMin=[]  SumDOutMax=[]  DifferentiatorOutMin=[]  DifferentiatorOutMax=[]  FilterDiffOutCoefMin=[]  FilterDiffOutCoefMax=[]  ReciprocalOutMin=[]  ReciprocalOutMax=[]  SumDenOutMin=[]  SumDenOutMax=[]  SumNumOutMin=[]  SumNumOutMax=[]  DivideOutMin=[]  DivideOutMax=[]  UdiffTsProdOutMin=[]  UdiffTsProdOutMax=[]  NTsProdOutMin=[]  NTsProdOutMax=[]  UintegralTsProdOutMin=[]  UintegralTsProdOutMax=[]  UngainTsProdOutMin=[]  UngainTsProdOutMax=[]  IntegratorContinuousStateAttributes=''  IntegratorStateMustResolveToSignalObject=off  IntegratorRTWStateStorageClass=Auto  FilterContinuousStateAttributes=''  FilterStateMustResolveToSignalObject=off  FilterRTWStateStorageClass=Auto  ParallelPVariant=InternalParameters  IdealPVariant=Disabled  IVariant=InternalParameters  DVariant=InternalParameters  IntegratorVariant=Continuous  SatVariant=Disabled  AWVariant=Passthrough  PCopyVariant=Disabled  TRVariant=Disabled  FdbkBlocksVariant=Forward  IdealPFdbkVariant=Disabled  SatFdbkVariant=Disabled  DerivativeFilterVariant=ContFilter  NVariant=InternalParameters  NCopyVariant=Disabled  FilterICVariant=InternalICsFilter  IntegratorICVariant=InternalICs  ExternalResetVariant=Disabled  TRSumVariant=Passthrough  SumFdbkVariant=Disabled  SumVariant=Sum_PID  TsampFilterVariant=InternalTs  TsampNgainVariant=Passthrough  TsampIntegralVariant=Passthrough  ExternalSaturationOutDataTypeStr=Inherit: Same as second input
  Scope : Scope
  Scope1 : Scope
  Scope2 : Scope
  Subsystem : Subsystem
  To Workspace : ToWorkspace  VariableName=g_force  SaveFormat=Timeseries  SampleTime=-1
      settings: Save2DSignal=2-D array (concatenate along first dimension)
  To Workspace1 : ToWorkspace  VariableName=r  SaveFormat=Timeseries  SampleTime=-1
  To Workspace2 : ToWorkspace  VariableName=F_control_minustau  SaveFormat=Timeseries  SampleTime=-1
  To Workspace3 : ToWorkspace  VariableName=v  SaveFormat=Timeseries  SampleTime=-1
  To Workspace4 : ToWorkspace  VariableName=a  SaveFormat=Timeseries  SampleTime=-1
  Transport Delay2 : TransportDelay  DelayTime=time_delay  TransDelayFeedthrough=on
  v^V : Outport
  a_pregyro : Outport  Port=2
  r : Outport  Port=3
  Fc(t-tau) : Outport  Port=4
  wires:
  Add5/1 -> Divide2/1
  PID Controller1/1 -> Gain/1
  a_kalman/1 -> Integrator8/1
  Gain/1 -> Mux/1
  Integrator8/1 -> v^V/1, To Workspace3/1, Integrator9/1  "v^V"
  Gain2/1 -> Mux/3
  F_aero^d/1 -> Add5/2
  r_trajectory/1 -> Add4/1
  PID Controller/1 -> Gain2/1  "F_z"
  Add4/1 -> Scope2/1, Demux/1
  Integrator9/1 -> r/1, To Workspace1/1  "r"
  Gain3/1 -> Transport Delay2/1, Scope/1  "F_c"
  Gain1/1 -> Mux/2
  Constant5/1 -> Divide2/2
  Demux/2 -> PID Controller2/1  "r_y"
  PID Controller2/1 -> Gain1/1
  r_Kalman/1 -> Add4/2
  Demux/1 -> PID Controller1/1  "r_x"
  Demux/3 -> PID Controller/1  "r_z"
  Divide/1 -> To Workspace/1
  Constant1/1 -> Divide/2
  Transport Delay2/1 -> Subsystem/1(Fc(t-tau)), To Workspace2/1  "Fc(t-tau)"
  Divide2/1 -> To Workspace4/1, a_pregyro/1, Scope1/1, Divide/1  "a"
  Fc_post_prop/1 -> Add5/1
  Mux/1 -> Gain3/1  "F_c"
  Subsystem/1(Fc_acc) -> Fc(t-tau)/1

== system LETS_GOOOOOO/Subsystem9 ==
  a_sensed : Inport
  position : Inport  Port=2
  Fc(t-tau) : Inport  Port=3
  Add : Sum  Inputs=+-
  Add1 : Sum  Inputs=+-
  Add2 : Sum  Inputs=+-
  Add3 : Sum
  GPS Model : MATLAB Function  TreatAsAtomicUnit=on
  Gain : Gain  Gain=0
  Gain1 : Gain
  Subsystem6 : Subsystem
  To Workspace : ToWorkspace  VariableName=GPS_error  SaveFormat=Timeseries  SampleTime=-1
  To Workspace1 : ToWorkspace  VariableName=Kal_tot  SaveFormat=Timeseries  SampleTime=-1
  To Workspace2 : ToWorkspace  VariableName=Kal_GPS  SaveFormat=Timeseries  SampleTime=-1
  Transpose : Math  Operator=transpose  SaturateOnIntegerOverflow=on
  r_kalman : Outport
  wires:
  GPS Model/1(newposition) -> Transpose/1, Gain1/1, Add2/2, Subsystem6/3(gps error)  "gps error"
  Fc(t-tau)/1 -> Subsystem6/1(Fc(t-tau))
  Subsystem6/1(r_kalman) -> Add2/1, Add1/2, Gain/1
  position/1 -> Add/1, Add1/1, GPS Model/1(position)
  a_sensed/1 -> Subsystem6/2(a_sensed)
  Add/1 -> To Workspace/1
  Add1/1 -> To Workspace1/1
  Add2/1 -> To Workspace2/1
  Transpose/1 -> Add/2
  Gain/1 -> Add3/1
  Gain1/1 -> Add3/2
  Add3/1 -> r_kalman/1

== system LETS_GOOOOOO/Wind gust1 ==
  Add : Sum  Inputs=+-
  Add1 : Sum  Inputs=+-
  Constant : Constant  Value=12.4
  Constant1 : Constant  Value=4.25
  Constant2 : Constant
  Constant3 : Constant  Value=0
  Constant4 : Constant  Value=0  VectorParams1D=off
  Mux : Mux  Inputs=3
  Product : Product
  Product1 : Product
  Sine Wave : Sin  Frequency=3*pi/T  SampleTime=0
  Sine Wave1 : Sin  Frequency=2*pi/T  Phase=pi/2  SampleTime=0
  V_tot : Outport
  wires:
  Constant/1 -> Add/1
  Constant1/1 -> Product/1
  Sine Wave/1 -> Product/2
  Constant2/1 -> Add1/1
  Sine Wave1/1 -> Add1/2
  Product/1 -> Product1/1
  Add1/1 -> Product1/2
  Product1/1 -> Add/2
  Add/1 -> Mux/2  "v_gust_y"
  Constant3/1 -> Mux/3  "v_gust_z"
  Constant4/1 -> Mux/1  "v_gust_x"
  Mux/1 -> V_tot/1

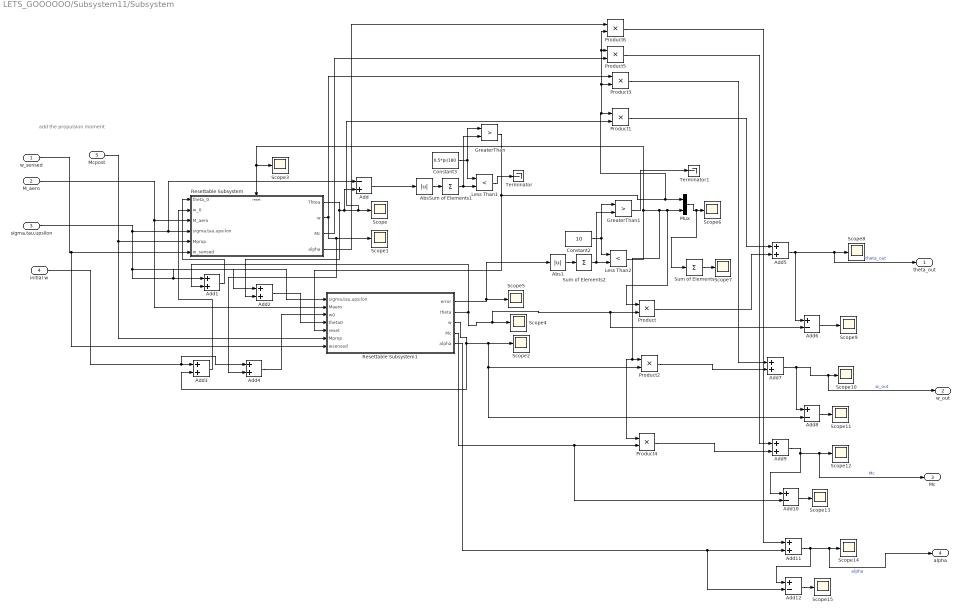
== system LETS_GOOOOOO/Subsystem11/Subsystem ==
  note: add the propulsion moment
  w_sensed : Inport
  M_aero : Inport  Port=2
  sigma,tau,upsilon : Inport  Port=3
  initial w : Inport  Port=4
  Mcpost : Inport  Port=5
  Abs : Abs
  Abs1 : Abs
  Add : Sum  Inputs=-+
  Add{1..5,7,9,11} (8 alike) : Sum
  Add{6,8,10,12} (4 alike) : Sum  Inputs=+-
  Constant2 : Constant  Value=10
  Constant3 : Constant  Value=0.5*pi/180
  GreaterThan : RelationalOperator  Operator=>  OutDataTypeStr=boolean  RndMeth=Simplest
  GreaterThan1 : RelationalOperator  Operator=>  OutDataTypeStr=boolean  RndMeth=Simplest
  Less Than1 : RelationalOperator  Operator=<  OutDataTypeStr=boolean  RndMeth=Simplest
  Less Than2 : RelationalOperator  Operator=<  OutDataTypeStr=boolean  RndMeth=Simplest
  Mux : Mux  Inputs=2
  Product{,1..6} (7 alike) : Product
  Resettable Subsystem : Subsystem  TreatAsAtomicUnit=on
  Resettable Subsystem1 : Subsystem  TreatAsAtomicUnit=on
  Scope{,1..15} (16 alike) : Scope
  Sum of Elements : Sum  Inputs=+
  Sum of Elements1 : Sum  Inputs=+
  Sum of Elements2 : Sum  Inputs=+
  Terminator : Terminator
  Terminator1 : Terminator
  theta_out : Outport
  w_out : Outport  Port=2
  Mc : Outport  Port=3
  alpha : Outport  Port=4
  wires:
  Add8/1 -> Scope11/1
  GreaterThan/1 -> Product6/2, Product5/1, Product3/2, Product1/1, Mux/1, Resettable Subsystem1/5(reset)
  Add6/1 -> Scope9/1
  Abs1/1 -> Sum of Elements2/1
  Product1/1 -> Add5/1
  Resettable Subsystem/2(w) -> Product3/1, Scope1/1, Add4/2
  Resettable Subsystem1/4(Mc) -> Add10/2, Product4/2
  Resettable Subsystem1/2(theta) -> Add6/2, Product/2, Scope4/1, Add1/2
  Resettable Subsystem1/5(alpha) -> Add12/2, Add11/2
  Resettable Subsystem/1(Thtea) -> Add2/2, Add/2, Product1/2, Scope/1
  Less Than2/1 -> Product2/1, Product4/1, Product/1, Mux/2, Scope3/1, Resettable Subsystem/Reset
  M_aero/1 -> Resettable Subsystem1/2(Maero), Resettable Subsystem/3(M_aero)
  Resettable Subsystem1/1(error) -> Abs1/1, Scope5/1
  Add11/1 -> Add12/1, alpha/1, Scope14/1  "alpha"
  Product2/1 -> Add7/2
  Constant2/1 -> GreaterThan1/1, Less Than2/1
  Resettable Subsystem1/3(w) -> Add3/2, Scope2/1, Add8/2, Product2/2
  Product3/1 -> Add7/1
  Add12/1 -> Scope15/1
  Abs/1 -> Sum of Elements1/1
  Add5/1 -> Add6/1, theta_out/1, Scope8/1  "theta_out"
  Add2/1 -> Resettable Subsystem1/4(theta0)
  Constant3/1 -> GreaterThan/1, Less Than1/1
  Sum of Elements1/1 -> Less Than1/2, GreaterThan/2
  Add3/1 -> Resettable Subsystem/2(w_0)
  sigma,tau,upsilon/1 -> Add2/1, Add1/1, Resettable Subsystem1/1(sigma,tau,upsilon), Add/1, Resettable Subsystem/4(sigma,tau,upsilon)
  Product5/1 -> Add9/1
  Resettable Subsystem/3(Mc) -> Product5/2
  Add7/1 -> Add8/1, w_out/1, Scope10/1  "w_out"
  Product6/1 -> Add11/1
  Add9/1 -> Add10/1, Mc/1, Scope12/1  "Mc"
  Add/1 -> Abs/1
  Add1/1 -> Resettable Subsystem/1(theta_0)
  Sum of Elements/1 -> Scope7/1
  Sum of Elements2/1 -> Less Than2/2, GreaterThan1/2
  Mcpost/1 -> Resettable Subsystem1/6(Mprop), Resettable Subsystem/5(Mprop)
  Mux/1 -> Sum of Elements/1, Scope6/1
  Resettable Subsystem/4(alpha) -> Product6/1
  Add4/1 -> Resettable Subsystem1/3(w0)
  initial w/1 -> Add4/1, Add3/1
  Product/1 -> Add5/2
  Add10/1 -> Scope13/1
  Product4/1 -> Add9/2
  GreaterThan1/1 -> Terminator1/1
  Less Than1/1 -> Terminator/1
  w_sensed/1 -> Resettable Subsystem1/7(wsensed), Resettable Subsystem/6(w_sensed)

== system LETS_GOOOOOO/Subsystem5/Subsystem ==
  F_c_d : Inport
  M_c_d : Inport  Port=2
  Demux8 : Demux  Outputs=3
  Demux9 : Demux  Outputs=3
  MATLAB Function : MATLAB Function  TreatAsAtomicUnit=on
  MATLAB Function6 : MATLAB Function  TreatAsAtomicUnit=on
  Mux23 : Mux
  Mux24 : Mux
  Mux9 : Mux  Inputs=3
  Terminator12 : Terminator
  To Workspace6 : ToWorkspace  VariableName=Fc_wanted  SaveFormat=Timeseries  SampleTime=-1
  To Workspace7 : ToWorkspace  VariableName=Ft_wanted  SaveFormat=Timeseries  SampleTime=-1
  To Workspace8 : ToWorkspace  VariableName=Fb_wanted  SaveFormat=Timeseries  SampleTime=-1
  Fb_wanted : Outport
  Ft_wanted : Outport  Port=2
  Fc_wanted : Outport  Port=3
  wires:
  Demux9/3 -> MATLAB Function6/3(M_z)
  Demux8/2 -> MATLAB Function6/1(F_y)
  Mux9/1 -> Fc_wanted/1, To Workspace6/1  "Fc_wanted"
  MATLAB Function/2(Ft2) -> Mux23/2  "Fb_wanted"
  Demux9/1 -> MATLAB Function6/2(M_x)
  MATLAB Function/3(Ft3) -> Mux23/3
  Demux9/2 -> MATLAB Function/1(My)
  MATLAB Function/8(Fb4) -> Mux24/4
  MATLAB Function6/1(F_c1) -> Mux9/1
  MATLAB Function/1(Ft1) -> Mux23/1  "Ft_wanted"
  Demux8/1 -> Terminator12/1
  Mux23/1 -> Ft_wanted/1, To Workspace7/1  "Ft_wanted"
  Mux24/1 -> Fb_wanted/1, To Workspace8/1  "Fb_wanted"
  MATLAB Function6/3(F_c3) -> Mux9/3
  MATLAB Function/5(Fb1) -> Mux24/1
  MATLAB Function/6(Fb2) -> Mux24/2
  MATLAB Function/7(Fb3) -> Mux24/3
  MATLAB Function/4(Ft4) -> Mux23/4
  Demux8/3 -> MATLAB Function/2(Fz)
  MATLAB Function6/2(F_c2) -> Mux9/2
  F_c_d/1 -> Demux8/1
  M_c_d/1 -> Demux9/1

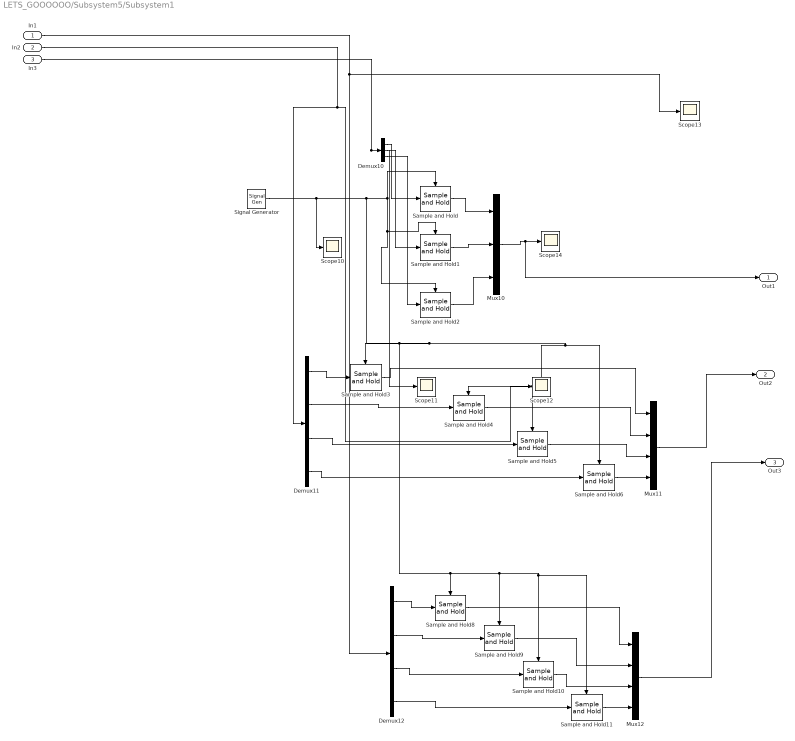
== system LETS_GOOOOOO/Subsystem5/Subsystem1 ==
  In1 : Inport
  In2 : Inport  Port=2
  In3 : Inport  Port=3
  Demux10 : Demux  Outputs=3
  Demux11 : Demux
  Demux12 : Demux
  Mux10 : Mux  Inputs=3
  Mux11 : Mux
  Mux12 : Mux
  Sample and Hold{,1..6,8..11} (11 alike) : dspsigops/Sample and Hold  trig=Rising edge  initCond=0  latchinput=off
  Scope{10..14} (5 alike) : Scope
  Signal Generator : SignalGenerator  WaveForm=square  Frequency=fprop  Units=rad/sec
  Out1 : Outport
  Out2 : Outport  Port=2
  Out3 : Outport  Port=3
  wires:
  Demux12/1 -> Sample and Hold8/1
  Demux11/1 -> Sample and Hold3/1
  Signal Generator/1 -> Scope10/1, Sample and Hold11/Trigger, Sample and Hold10/Trigger, Sample and Hold9/Trigger, Sample and Hold8/Trigger, Sample and Hold4/Trigger, Sample and Hold5/Trigger, Sample and Hold6/Trigger, Sample and Hold3/Trigger, Sample and Hold/Trigger, Sample and Hold2/Trigger, Sample and Hold1/Trigger
  In2/1 -> Scope12/1, Demux11/1
  In3/1 -> Scope11/1, Demux10/1
  Demux10/3 -> Sample and Hold2/1
  Sample and Hold10/1 -> Mux12/3
  Sample and Hold/1 -> Mux10/1
  Demux12/4 -> Sample and Hold11/1
  Sample and Hold6/1 -> Mux11/4
  Demux10/1 -> Sample and Hold/1
  Mux10/1 -> Out1/1, Scope14/1
  Demux12/3 -> Sample and Hold10/1
  Sample and Hold8/1 -> Mux12/1
  Sample and Hold3/1 -> Mux11/1
  Sample and Hold5/1 -> Mux11/3
  Sample and Hold1/1 -> Mux10/2
  Sample and Hold11/1 -> Mux12/4
  In1/1 -> Scope13/1, Demux12/1
  Demux10/2 -> Sample and Hold1/1
  Demux11/2 -> Sample and Hold4/1
  Sample and Hold2/1 -> Mux10/3
  Sample and Hold4/1 -> Mux11/2
  Sample and Hold9/1 -> Mux12/2
  Demux11/3 -> Sample and Hold5/1
  Mux12/1 -> Out3/1
  Demux12/2 -> Sample and Hold9/1
  Demux11/4 -> Sample and Hold6/1
  Mux11/1 -> Out2/1

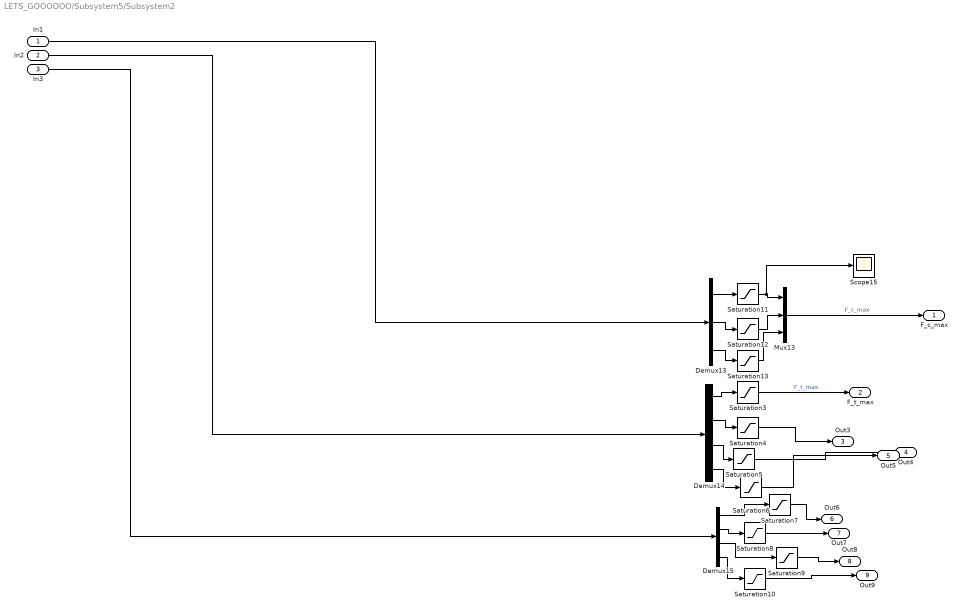
== system LETS_GOOOOOO/Subsystem5/Subsystem2 ==
  In1 : Inport
  In2 : Inport  Port=2
  In3 : Inport  Port=3
  Demux13 : Demux  Outputs=3
  Demux14 : Demux
  Demux15 : Demux
  Mux13 : Mux  Inputs=3
  Saturation10 : Saturate  UpperLimit=Fb4_u  LowerLimit=Fb4_l
  Saturation11 : Saturate  UpperLimit=Fc1_u  LowerLimit=Fc1_l
  Saturation12 : Saturate  UpperLimit=Fc2_u  LowerLimit=Fc2_l
  Saturation13 : Saturate  UpperLimit=Fc3_u  LowerLimit=Fc3_l
  Saturation3 : Saturate  UpperLimit=Ft1_u  LowerLimit=Ft1_l
  Saturation4 : Saturate  UpperLimit=Ft2_u  LowerLimit=Ft2_l
  Saturation5 : Saturate  UpperLimit=Ft3_u  LowerLimit=Ft3_l
  Saturation6 : Saturate  UpperLimit=Ft4_u  LowerLimit=Ft4_l
  Saturation7 : Saturate  UpperLimit=Fb1_u  LowerLimit=Fb1_l
  Saturation8 : Saturate  UpperLimit=Fb2_u  LowerLimit=Fb2_l
  Saturation9 : Saturate  UpperLimit=Fb3_u  LowerLimit=Fb3_l
  Scope15 : Scope
  F_c_max : Outport
  F_t_max : Outport  Port=2
  Out3 : Outport  Port=3
  Out4 : Outport  Port=4
  Out5 : Outport  Port=5
  Out6 : Outport  Port=6
  Out7 : Outport  Port=7
  Out8 : Outport  Port=8
  Out9 : Outport  Port=9
  wires:
  Saturation11/1 -> Scope15/1, Mux13/1
  Demux13/2 -> Saturation12/1
  Saturation10/1 -> Out9/1
  Demux13/3 -> Saturation13/1
  Demux14/1 -> Saturation3/1
  Demux14/4 -> Saturation6/1
  In3/1 -> Demux15/1
  Demux14/3 -> Saturation5/1
  Demux13/1 -> Saturation11/1
  Saturation13/1 -> Mux13/3
  In1/1 -> Demux13/1
  Demux15/1 -> Saturation7/1
  Demux15/2 -> Saturation8/1
  Demux15/3 -> Saturation9/1
  Saturation12/1 -> Mux13/2
  Demux15/4 -> Saturation10/1
  Demux14/2 -> Saturation4/1
  Saturation9/1 -> Out8/1
  Saturation5/1 -> Out4/1
  In2/1 -> Demux14/1
  Saturation4/1 -> Out3/1
  Saturation7/1 -> Out6/1
  Mux13/1 -> F_c_max/1  "F_c_max"
  Saturation6/1 -> Out5/1
  Saturation3/1 -> F_t_max/1  "F_t_max"
  Saturation8/1 -> Out7/1

== system LETS_GOOOOOO/Subsystem5/Subsystem3 ==
  In1 : Inport
  In2 : Inport  Port=2
  In3 : Inport  Port=3
  Ft3 : Inport  Port=4
  Ft4 : Inport  Port=5
  Fb1 : Inport  Port=6
  In7 : Inport  Port=7
  Fb3 : Inport  Port=8
  In9 : Inport  Port=9
  Constant23 : Constant  Value=0
  Demux16 : Demux  Outputs=3
  MATLAB Function7 : MATLAB Function  TreatAsAtomicUnit=on
  MATLAB Function8 : MATLAB Function  TreatAsAtomicUnit=on
  MATLAB Function9 : MATLAB Function  TreatAsAtomicUnit=on
  Mux : Mux
  Mux1 : Mux
  Mux16 : Mux  Inputs=3
  Mux17 : Mux  Inputs=3
  To Workspace : ToWorkspace  VariableName=Fc  SaveFormat=Timeseries  SampleTime=-1
  To Workspace1 : ToWorkspace  VariableName=Ft  SaveFormat=Timeseries  SampleTime=-1
  To Workspace2 : ToWorkspace  VariableName=Fb  SaveFormat=Timeseries  SampleTime=-1
  Out1 : Outport
  Mc(t-tau)_actual : Outport  Port=2
  wires:
  Demux16/2 -> MATLAB Function8/2(F_c2)
  In9/1 -> Mux1/4, MATLAB Function9/8(Fb4)
  In3/1 -> Mux/2, MATLAB Function9/2(Ft2)
  MATLAB Function7/1(F_z) -> Mux16/3  "Fz_actual"
  In1/1 -> Demux16/1, To Workspace/1
  Fb3/1 -> Mux1/3, MATLAB Function9/7(Fb3)
  MATLAB Function9/1(F1) -> MATLAB Function7/1(F1)
  Ft3/1 -> Mux/3, MATLAB Function9/3(Ft3)
  MATLAB Function8/1(F_y) -> Mux16/2  "Fy_actual"
  Fb1/1 -> Mux1/1, MATLAB Function9/5(Fb1)
  MATLAB Function8/3(M_z) -> Mux17/3  "M_z_acc"
  MATLAB Function7/2(M_y) -> Mux17/2  "M_y_acc"
  Mux17/1 -> Mc(t-tau)_actual/1  "Mc(t-tau)_actual"
  Ft4/1 -> Mux/4, MATLAB Function9/4(Ft4)
  MATLAB Function8/2(M_x) -> Mux17/1  "M_x_acc"
  In7/1 -> Mux1/2, MATLAB Function9/6(Fb2)
  MATLAB Function9/3(F3) -> MATLAB Function7/3(F3)
  Demux16/1 -> MATLAB Function8/1(F_c1)
  Constant23/1 -> Mux16/1  "Fx_actual"
  In2/1 -> Mux/1, MATLAB Function9/1(Ft1)
  MATLAB Function9/2(F2) -> MATLAB Function7/2(F2)
  Mux1/1 -> To Workspace2/1
  Demux16/3 -> MATLAB Function8/3(F_c3)
  Mux/1 -> To Workspace1/1
  Mux16/1 -> Out1/1

== system LETS_GOOOOOO/Subsystem5/Subsystem4 ==
  TVd : Inport
  In2 : Inport  Port=2
  Constant24 : Constant  Value=[0;1;1]
  Matrix Multiply3 : Product  Multiplication=Matrix(*)
  Product5 : Product
  Fc(t-tau)_actual : Outport
  Fc(t-tau)_actual1 : Outport  Port=2
  wires:
  Matrix Multiply3/1 -> Fc(t-tau)_actual1/1, Product5/2  "Fc(t-tau)_actual"
  Constant24/1 -> Product5/1
  TVd/1 -> Matrix Multiply3/1
  Product5/1 -> Fc(t-tau)_actual/1  "Fc(t-tau)_actual"
  In2/1 -> Matrix Multiply3/2

== system LETS_GOOOOOO/Subsystem8/Subsystem ==
  Fc(t-tau) : Inport
  Abs : Abs
  Add : Sum  Inputs=+++
  Add1 : Sum
  Add2 : Sum
  Constant : Constant  Value=F_tot_max
  Constant1 : Constant  Value=10^(-8)
  Demux1 : Demux  Outputs=3
  Divide1 : Product  Inputs=*/
  Gain4 : Gain  Gain=F_tot_max
  GreaterThan : RelationalOperator  Operator=>  OutDataTypeStr=boolean  RndMeth=Simplest
  Less Than : RelationalOperator  Operator=<  OutDataTypeStr=boolean  RndMeth=Simplest
  Product : Product
  Product1 : Product
  Scope{,1..2,4} (4 alike) : Scope
  Square : Math  Operator=square  SaturateOnIntegerOverflow=on
  Square Root : Sqrt  SaturateOnIntegerOverflow=on
  Square1 : Math  Operator=square  SaturateOnIntegerOverflow=on
  Square2 : Math  Operator=square  SaturateOnIntegerOverflow=on
  Sum of Elements : Sum  Inputs=+
  Fc_acc : Outport
  wires:
  Gain4/1 -> Product/2
  Divide1/1 -> Scope4/1, Gain4/1
  Demux1/1 -> Square/1
  Abs/1 -> Sum of Elements/1
  Fc(t-tau)/1 -> Product1/1, Demux1/1, Divide1/1, Abs/1
  Square/1 -> Add/1
  Sum of Elements/1 -> Add2/1
  Demux1/3 -> Square2/1
  Square2/1 -> Add/3
  Square1/1 -> Add/2
  Demux1/2 -> Square1/1
  Add/1 -> Square Root/1
  Square Root/1 -> Less Than/1, Scope1/1, GreaterThan/1
  Constant/1 -> GreaterThan/2, Less Than/2
  GreaterThan/1 -> Scope2/1, Product/1
  Less Than/1 -> Product1/2
  Product/1 -> Add1/2
  Product1/1 -> Add1/1
  Add1/1 -> Fc_acc/1, Scope/1
  Constant1/1 -> Add2/2
  Add2/1 -> Divide1/2

== system LETS_GOOOOOO/Subsystem9/Subsystem6 ==
  Fc(t-tau) : Inport
  a_sensed : Inport  Port=2
  gps error : Inport  Port=3
  Constant8 : Constant  Value=0
  Demux2 : Demux  Outputs=6
  Integrator1 : Integrator  InitialCondition=v_0
  Kalman Filter : ctrlSharedLib/Kalman Filter  TimeDomain=Continuous-Time  UseCurrentEstimator=on  ModelSource=Individual A, B, C, D matrices  ModelSourceVariable=ss(0.95,1,1,0,1)  A=A_kal  B=B_kal  C=C_kal  D=D_kal  NumberOfStates=1  NumberOfInputs=1  NumberOfOutputs=1  InitialEstimateSource=Dialog  X0=[0;0;0;0;0;0]  P0=10  UseK=off  UseGH=off  NumberOfProcessNoiseInputs=1  G=1  TimeInvariantG=on  H=0  TimeInvariantH=on  Q=0.05  TimeInvariantQ=on  R=1  TimeInvariantR=on  N=0  TimeInvariantN=on  AddInputPort=on  AddEnablePort=off  OutputEstimatedY=off  OutputP=off  Ts=-1
  Mux1 : Mux
  Mux3 : Mux  Inputs=3
  Mux4 : Mux  Inputs=2
  Terminator : Terminator
  Terminator2 : Terminator
  Terminator3 : Terminator
  Transpose : Math  Operator=transpose  SaturateOnIntegerOverflow=on
  r_kalman : Outport
  wires:
  Integrator1/1 -> Mux4/2  "v_sensed"
  Demux2/2 -> Mux3/2
  Kalman Filter/1 -> Demux2/1
  Constant8/1 -> Mux1/1, Mux1/3, Mux1/2
  Transpose/1 -> Mux4/1  "r_sensed"
  Mux1/1 -> Kalman Filter/1
  Demux2/4 -> Terminator/1
  Demux2/1 -> Mux3/1
  Demux2/3 -> Mux3/3
  Mux4/1 -> Kalman Filter/2
  Demux2/5 -> Terminator3/1
  Demux2/6 -> Terminator2/1
  Fc(t-tau)/1 -> Mux1/4
  Mux3/1 -> r_kalman/1  "r_kalman"
  gps error/1 -> Transpose/1
  a_sensed/1 -> Integrator1/1
